simulink model "car_suspension_control101"  (R2023a)
settings: Solver=ode45  StartTime=0.0  StopTime=t_stop  RelTol=1e-3  EnableMultiTasking=on
values from neighbouring files (symbols this model uses):
  M = 1000    [simulink_openloop_model_control101_script.m]    (also in simulink_openloop_modelb_control101_script.m; simulink_openloop_modelc_control101_script.m; simulink_openloop_modeld_control101_script.m)
undefined symbols (not defined in the file or in its folder): b, k1, k2
settings Model: Creator=uos  LastModifiedBy=Anthony Rossiter
settings SolverCC: AlgebraicLoopSolver=TrustRegion
settings DataIOCC: LimitDataPoints=on  SaveFormat=Array  SignalLoggingSaveFormat=ModelDataLogs  ReturnWorkspaceOutputs=off
settings OptimizationCC: BooleanDataType=off  ExpressionDepthLimit=2147483647  LifeSpan=inf
settings DebuggingCC: SaveWithParameterizedLinksMsg=none  UnderspecifiedInitializationDetection=Classic  MergeDetectMultiDrivingBlocksExec=none  SignalResolutionControl=TryResolveAllWithWarning  MultiTaskDSMMsg=warning  MultiTaskCondExecSysMsg=none  FcnCallInpInsideContextMsg=warning  UnconnectedInputMsg=warning  UnconnectedOutputMsg=warning  UnconnectedLineMsg=warning  StateNameClashWarn=warning  SFUnexpectedBacktrackingDiag=warning  SFNoUnconditionalDefaultTransitionDiag=warning  SFExecutionAtInitializationDiag=none  ArithmeticOperatorsInVariantConditions=warning
settings HardwareCC: ProdBitPerPointer=32  ProdBitPerSizeT=32  ProdBitPerPtrDiffT=32  ProdLargestAtomicFloat=None  ProdIntDivRoundTo=Undefined  ProdEndianess=Unspecified  ProdWordSize=32  ProdHWDeviceType=32-bit Generic  TargetUnknown=on
settings ModelReferenceCC: EnableRefExpFcnMdlSchedulingChecks=on  PropagateSignalLabelsOutOfModel=off
settings SFSimCC: SimUseLocalCustomCode=off  CustomCodeUndefinedFunction=UseInterfaceOnly
settings RTWCC: RTWUseLocalCustomCode=off  DLArmComputeVersion=19.05
settings CodeAppCC: StateflowObjectComments=on
settings GRTTargetCC: TargetLangStandard=C89/C90 (ANSI)  CombineOutputUpdateFcns=off  GRTInterface=on
settings ConfigComp: CovMetricSettings=dw  CovSaveCumulativeToWorkspaceVar=on  CovSaveSingleToWorkspaceVar=on  CovExternalEMLEnable=off

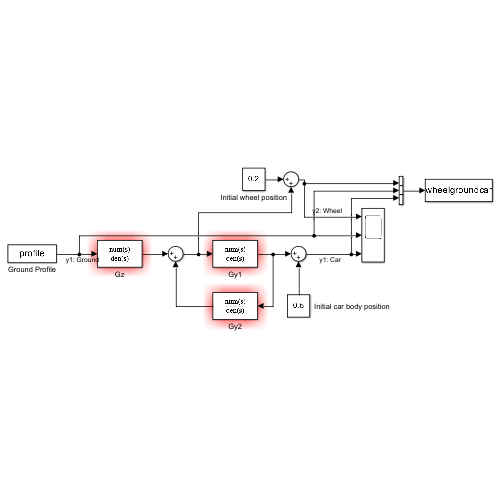
[thumbnail: Simulink's stored preview of the top-level diagram]
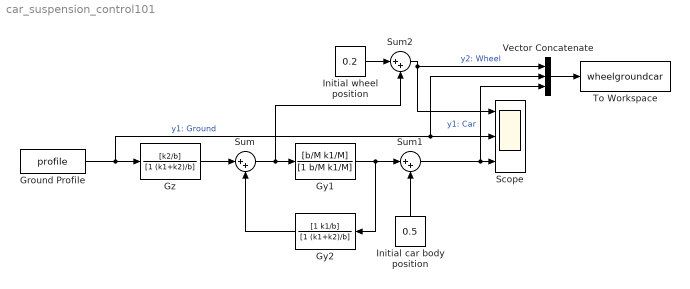
== system car_suspension_control101 ==
  Ground Profile : FromWorkspace  VariableName=profile  Interpolate=off  ZeroCross=off  OutputAfterFinalValue=Holding final value
  Gy1 : TransferFcn  Numerator=[b/M k1/M]  Denominator=[1 b/M k1/M]
  Gy2 : TransferFcn  Numerator=[1 k1/b]  Denominator=[1 (k1+k2)/b]
  Gz : TransferFcn  Numerator=[k2/b]  Denominator=[1 (k1+k2)/b]
  Initial car body position : Constant  Value=0.5
  Initial wheel position : Constant  Value=0.2
  Scope : Scope  NumInputPorts=3
  Sum : Sum  Inputs=|++  InputSameDT=on  SaturateOnIntegerOverflow=on  OutDataTypeStr=Inherit: Same as first input
  Sum1 : Sum  Inputs=|++  InputSameDT=on  SaturateOnIntegerOverflow=on  OutDataTypeStr=Inherit: Same as first input
  Sum2 : Sum  Inputs=|++  InputSameDT=on  SaturateOnIntegerOverflow=on  OutDataTypeStr=Inherit: Same as first input
  To Workspace : ToWorkspace  VariableName=wheelgroundcar  SaveFormat=Structure With Time  SampleTime=-1
  Vector Concatenate : Concatenate  NumInputs=3
  wires:
  Ground Profile/1 -> Vector Concatenate/2, Scope/2, Gz/1  "y1: Ground"
  Gz/1 -> Sum/1
  Sum/1 -> Gy1/1, Sum2/2
  Gy1/1 -> Sum1/1, Gy2/1
  Gy2/1 -> Sum/2
  Initial car body position/1 -> Sum1/2
  Initial wheel position/1 -> Sum2/1
  Sum1/1 -> Vector Concatenate/3, Scope/3  "y1: Car"
  Sum2/1 -> Scope/1, Vector Concatenate/1  "y2: Wheel"
  Vector Concatenate/1 -> To Workspace/1
